simulink model "ballistic_model"  (R2022a)
settings: Solver=VariableStepAuto  StartTime=0.0  StopTime=t_final  MaxStep=t_step_size  RelTol=1e-3
values from neighbouring files (symbols this model uses):
  g = 9.81    [ballistic_model_solver.m]    (also in point_of_interest_calc.m; solver.m)
  ground_level = -1    [ballistic_model_solver.m]    (also in point_of_interest_calc.m)
  m = 0.032    [ballistic_model_solver.m]    (also in point_of_interest_calc.m; solver.m = 2)
  medium_viscosity = 0    [ballistic_model_solver.m]    (also in point_of_interest_calc.m)
  radius_projectile = 16.8 / 2    (= 8.4)    [ballistic_model_solver.m]    (also in point_of_interest_calc.m)
  vx = limiting_v * cosd(aor)    [ballistic_model_solver.m]    (also in point_of_interest_calc.m)
  vy = limiting_v * sind(aor)    [ballistic_model_solver.m]    (also in point_of_interest_calc.m)
libraries: simulink x1
settings Model: Creator=dhiro  LastModifiedBy=dhiro

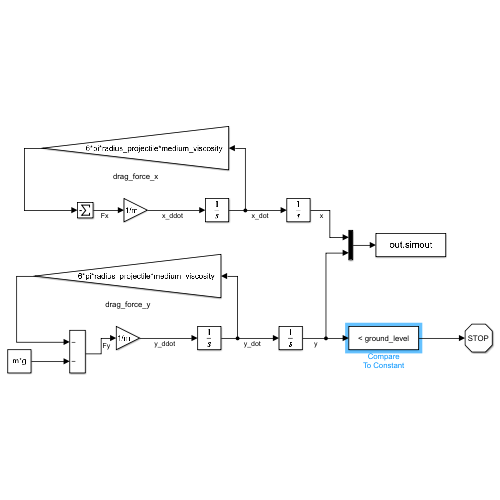
[thumbnail: Simulink's stored preview of the top-level diagram]
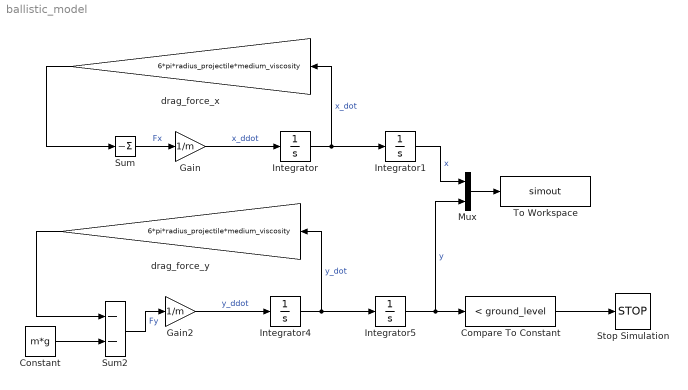
== system ballistic_model ==
  Compare To Constant : simulink/Logic and Bit Operations/Compare To Constant  relop=<  const=ground_level  OutDataTypeStr=boolean
  Constant : Constant  Value=m*g
  Gain : Gain  Gain=1/m
  Gain2 : Gain  Gain=1/m
  Integrator : Integrator  InitialCondition=vx
  Integrator1 : Integrator
  Integrator4 : Integrator  InitialCondition=vy
  Integrator5 : Integrator
  Mux : Mux  Inputs=2
  Stop Simulation : Stop
  Sum : Sum  Inputs=-
  Sum2 : Sum  Inputs=--
  To Workspace : ToWorkspace  VariableName=simout  SaveFormat=Timeseries  SampleTime=-1
  drag_force_x : Gain  Gain=6*pi*radius_projectile*medium_viscosity
  drag_force_y : Gain  Gain=6*pi*radius_projectile*medium_viscosity
  wires:
  Sum/1 -> Gain/1  "Fx"
  Gain/1 -> Integrator/1  "x_ddot"
  Integrator/1 -> drag_force_x/1, Integrator1/1  "x_dot"
  drag_force_x/1 -> Sum/1
  Integrator4/1 -> Integrator5/1, drag_force_y/1  "y_dot"
  Gain2/1 -> Integrator4/1  "y_ddot"
  drag_force_y/1 -> Sum2/1
  Sum2/1 -> Gain2/1  "Fy"
  Constant/1 -> Sum2/2
  Integrator1/1 -> Mux/1  "x"
  Integrator5/1 -> Compare To Constant/1, Mux/2  "y"
  Mux/1 -> To Workspace/1
  Compare To Constant/1 -> Stop Simulation/1
